simulink model "sm_boom_lift_crawler_abstract"  (R2026a)
settings: Solver=ode23t  StopTime=operator_seq.StopTime  FixedStep=2e-2  MaxStep=2  AbsTol=1e-3
PreLoadFcn:
  | sm_boom_lift_crawler_settest('full test')
StartFcn:
  | tic;
StopFcn:
  | Elapsed_Sim_Time = toc;
  | %disp(['Elapsed Sim Time = ' num2str(Elapsed_Sim_Time)]);
undefined symbols (not defined in the file): BasketR, Boom, Chassis, Extend, Jib, LevelM, LevelS, Lift, operator_seq, OutFL, OutFR, OutRL, OutRR, Tilt, TrackL, TrackR, Turret
libraries: sm_boom_lift_crawler_lib x14, sm_lib x2, sm_boom_lift_crawler_lib_control x1, sm_boom_lift_crawler_lib_lift x1, nesl_utility x1
Description:
  | Boom Lift Crawler with Abstract Actuator Models and Controller
  | 
  | Copyright 2020-2026 The MathWorks, Inc.
settings Model: PacingRate=0.100000  Creator=smiller  LastModifiedBy=smiller
settings DataIOCC: SignalLoggingName=logsout_sm_boom_lift_crawler
settings SimscapeCC: SimscapeNominalValues="[{\"value\":\"1\",\"unit\":\"A\"},{\"value\":\"nomval_psi\",\"unit\":\"psi\"},{\"value\":\"1\",\"unit\":\"cm^2\"},{\"value\":\"nomval_cmv3_s\",\"unit\":\"cm^3/s\"},{\"value\":\"1\",\"unit\":\"kJ/kg\"},{\"value\":\"1\",\"unit\":\"kW\"},{\"value\":\"1\",\"unit\":\"l\"},{\"value\":\"nomval_N\",\"unit\":\"N\"},{\"value\":\"nomval_Nm\",\"unit\":\"N*m\"},{\"value\":\"1\",\"unit\":\"V\"}]"  SimscapeLogName=simlog_sm_boom_lift_crawler  SimscapeLogLimitData=off  SimscapeLogDataHistory=5000.0  SimscapeOperatingPoint=op_hold15Sec_FULL
settings DiagnosticsConfigSet: SimMechanicsConflictingReferenceFrames=none  SimMechanicsRigidlyBoundBlock=none
settings ExplorerConfigSet: InternalSimMechanicsExplorerSettings="<ExplorerConfiguration><canonicalview>default</canonicalview><AnimationSetting><BasePlaybackSpeed>1.0</BasePlaybackSpeed><PlaybackSpeedFactor>4.0</PlaybackSpeedFactor></AnimationSetting><TilePanel><TileInfo><Tiles Columns=\"2\" Count=\"3\" Rows=\"2\"><Column Weight=\"0.4762\"/><Column Weight=\"0.5238\"/><Row Weight=\"0.5\"/><Row Weight=\"0.5\"/><Tile Height=\"1\" Width=\"1\" X=\"0\" Y=\"0\"/><Tile Height=\"1\" Width=\"1\" X=\"0\" Y=\"1\"/><Tile Height=\"2\" Width=\"1\" X=\"1\" Y=\"0\"/></Tiles></TileInfo><SceneInfo><SceneViewer><BGColor><R>1</R><G>1</G><B>1</B></BGColor><Camera><DoPerspective>off</DoPerspective><Position><X>0.0516797948744336932</X><Y>0.487181813254666363</Y><Z>16.9590725690521751</Z></Position><Center><X>0.0516797948744336932</X><Y>0.487181813254666363</Y><Z>1.03715866228651166</Z></Center><Up><X>0.999999952444677764</X><Y>0.000308400133790180664</Y><Z>0</Z></Up><ViewLimDist>1</ViewLimDist><YLim>2.49915112509375037</YLim><XLim>5.22931621973398197</XLim></Camera></SceneViewer><SceneViewer><BGColor><R>1</R><G>1</G><B>1</B></BGColor><Camera><DoPerspective>off</DoPerspective><Position><X>-11.4895183893373876</X><Y>4.05584925644575378e-08</Y><Z>1.89929114001093824</Z></Position><Center><X>-2.67728871072847596e-07</X><Y>4.05584925644575378e-08</Y><Z>1.89929114001093824</Z></Center><Up><X>0</X><Y>0</Y><Z>1</Z></Up><ViewLimDist>1</ViewLimDist><YLim>2.64934859154929603</YLim><XLim>5.54359495206533381</XLim></Camera></SceneViewer><SceneViewer><BGColor><R>1</R><G>1</G><B>1</B></BGColor><Camera><DoPerspective>on</DoPerspective><Position><X>0.00209723334754329926</X><Y>1.29823210500621533</Y><Z>0.569634199895673765</Z></Position><Center><X>0.00166989381543739923</X><Y>2.29823093449923377</Y><Z>0.568165052688056504</Z></Center><Up><X>-0.00271868050236136628</X><Y>0.00146798011384896131</Y><Z>0.999995226893964473</Z></Up><ViewLimDist>1</ViewLimDist><YLim>0.466307658154998583</YLim><XLim>0.530158914250911217</XLim></Camera></SceneViewer></SceneInfo></TilePanel><MechEditorPanel><Cameras><Camera><Id>Camera8</Id><Value><Name>Extend_Knuckle</Name><NativeCamera><PositionTrackingFeature>Lift.Boom.Arms.Telescope.Extend_Cylinder.Transform_Camera_Extend_Knuckle.F</PositionTrackingFeature><CenterTrackingFeature>Lift.Boom.Arms.Telescope.Extend_Cylinder.Transform_Camera_Extend_Knuckle.F</CenterTrackingFeature><UpVectorTrackingFeature>Lift.Boom.Arms.Telescope.Extend_Cylinder.Transform_Camera_Extend_Knuckle.F</UpVectorTrackingFeature><CenterTrackingOrigin>off</CenterTrackingOrigin><CenterTrackingDirection>-X</CenterTrackingDirection><UpVectorTrackingDirection>-Y</UpVectorTrackingDirection></NativeCamera></Value></Camera><Camera><Id>Camera9</Id><Value><Name>Extend_Basket</Name><NativeCamera><PositionTrackingFeature>Lift.Boom.Arms.Telescope.Extend_Cylinder.Transform_Camera_Extend_Basket.F</PositionTrackingFeature><CenterTrackingFeature>Lift.Boom.Arms.Telescope.Extend_Cylinder.Transform_Camera_Extend_Basket.F</CenterTrackingFeature><UpVectorTrackingFeature>Lift.Boom.Arms.Telescope.Extend_Cylinder.Transform_Camera_Extend_Basket.F</UpVectorTrackingFeature><CenterTrackingOrigin>off</CenterTrackingOrigin><CenterTrackingDirection>+X</CenterTrackingDirection><UpVectorTrackingDirection>+Y</UpVectorTrackingDirection></NativeCamera></Value></Camera><Camera><Id>Camera10</Id><Value><Name>Basket_Rotate</Name><NativeCamera><PositionTrackingFeature>Lift.Boom.Basket.Basket_Rotate.Bracket.Reference_Camera_Basket_Rotate_L.R</PositionTrackingFeature><CenterTrackingFeature>Lift.Boom.Basket.Basket_Rotate.Bracket.Reference_Camera_Basket_Rotate_L.R</CenterTrackingFeature><UpVectorTrackingFeature>Mech_Config.World.W</UpVectorTrackingFeature><CenterTrackingOrigin>off</CenterTrackingOrigin><CenterTrackingDirection>-X</CenterTrackingDirection><UpVectorTrackingDirection>+Z</UpVectorTrackingDirection></NativeCamera></Value></Camera><Camera><Id>Camera11</Id><Value><Name>Tilt_Knuckle</Name><NativeCamera><PositionTrackingFeature>Lift.Boom.Arms.Tower.Upper_Knuckle.Reference_Knuckle_Cam.R</PositionTrackingFeature><CenterTrackingFeature>Lift.Boom.Arms.Tower.Upper_Knuckle.Reference_Knuckle_Cam.R</CenterTrackingFeature><UpVectorTrackingFeature>Mech_Config.World.W</UpVectorTrackingFeature><CenterTrackingOrigin>off</CenterTrackingOrigin><CenterTrackingDirection>+Z</CenterTrackingDirection><UpVectorTrackingDirection>+Z</UpVectorTrackingDirection></NativeCamera></Value></Camera><Camera><Id>Camera12</Id><Value><Name>Full Test</Name><NativeCamera><PositionKeyframeSet><Keyframe><Time>0</Time><Value><X>-12.242458171438994</X><Y>-0.1433452642095574</Y><Z>4.1505972342390427</Z></Value></Keyframe><Keyframe><Time>69.026826430124729</Time><Value><X>-14.974593328379619</X><Y>0.0056652615564253064</Y><Z>5.3389029552684786</Z></Value></Keyframe><Keyframe><Time>110.29539843687829</Time><Value><X>-21.00761369699504</X><Y>-0.0057417156870510078</Y><Z>8.0689402037867488</Z></Value></Keyframe><Keyframe><Time>140.70430157635164</Time><Value><X>-31.272784439198116</X><Y>-2.5583130214499052e-10</Y><Z>12.723321478963756</Z></Value></Keyframe><Keyframe><Time>181.77628976806102</Time><Value><X>-31.272784439198116</X><Y>-2.5583130214499052e-10</Y><Z>12.723321478963756</Z></Value></Keyframe><Keyframe><Time>208.0087867386398</Time><Value><X>-23.351505250921551</X><Y>-2.5583182919801497e-10</Y><Z>9.1371534281977738</Z></Value></Keyframe><Keyframe><Time>243.06358572448306</Time><Value><X>-16.577121762622586</X><Y>-2.5583144573665537e-10</Y><Z>6.0702143126734844</Z></Value></Keyframe><Keyframe><Time>273.3415757110605</Time><Value><X>-16.577121762622586</X><Y>-2.5583144573665537e-10</Y><Z>6.0702143126734844</Z></Value></Keyframe><Keyframe><Time>321.2447002217541</Time><Value><X>-13.690590902490033</X><Y>0.01787769923724114</Y><Z>4.7891626503614262</Z></Value></Keyframe><Keyframe><Time>350</Time><Value><X>-13.690590902490033</X><Y>0.01787769923724114</Y><Z>4.7891626503614262</Z></Value></Keyframe></PositionKeyframeSet><CenterKeyframeSet><Keyframe><Time>0</Time><Value><X>-4.621228999686064</X><Y>-0.1433452642095574</Y><Z>4.1505972342390436</Z></Value></Keyframe><Keyframe><Time>69.026826430124729</Time><Value><X>-0.17395018713353672</X><Y>0.0056652615564253064</Y><Z>5.3389029552684786</Z></Value></Keyframe><Keyframe><Time>110.29539843687829</Time><Value><X>-9.0038066291239502</X><Y>-0.0057417156870549491</Y><Z>8.0689402037867524</Z></Value></Keyframe><Keyframe><Time>140.70430157635164</Time><Value><X>-14.136391845814327</X><Y>-2.5583979379462107e-10</Y><Z>12.72332147896376</Z></Value></Keyframe><Keyframe><Time>181.77628976806102</Time><Value><X>-2.3429975002054775</X><Y>-2.5584563781180217e-10</Y><Z>12.723321478963761</Z></Value></Keyframe><Keyframe><Time>208.0087867386398</Time><Value><X>-10.17575261115104</X><Y>-2.5583801743778167e-10</Y><Z>9.1371534281977755</Z></Value></Keyframe><Keyframe><Time>243.06358572448306</Time><Value><X>-0.54476849060194255</X><Y>-2.5583897563257738e-10</Y><Z>6.0702143126734844</Z></Value></Keyframe><Keyframe><Time>273.3415757110605</Time><Value><X>-0.11057247639663359</X><Y>-2.5583917956089291e-10</Y><Z>6.0702143126734844</Z></Value></Keyframe><Keyframe><Time>321.2447002217541</Time><Value><X>-5.3452949964231387</X><Y>0.017877699237237366</Y><Z>4.7891626503614253</Z></Value></Keyframe><Keyframe><Time>350</Time><Value><X>-5.3452949964231387</X><Y>0.017877699237237366</Y><Z>4.7891626503614253</Z></Value></Keyframe></CenterKeyframeSet><UpVectorKeyframeSet><Keyframe><Time>0</Time><Value><X>0</X><Y>0</Y><Z>1</Z></Value></Keyframe><Keyframe><Time>69.026826430124729</Time><Value><X>0</X><Y>0</Y><Z>1</Z></Value></Keyframe><Keyframe><Time>110.29539843687829</Time><Value><X>0</X><Y>0</Y><Z>1</Z></Value></Keyframe><Keyframe><Time>140.70430157635164</Time><Value><X>0</X><Y>0</Y><Z>1</Z></Value></Keyframe><Keyframe><Time>181.77628976806102</Time><Value><X>-2.0731981129868445e-16</X><Y>1.0273382740432149e-31</Y><Z>1</Z></Value></Keyframe><Keyframe><Time>208.0087867386398</Time><Value><X>1.4663775813922931e-57</X><Y>2.9591920320379324e-42</Y><Z>1</Z></Value></Keyframe><Keyframe><Time>243.06358572448306</Time><Value><X>1.3898401336634517e-57</X><Y>2.9591920320379324e-42</Y><Z>1</Z></Value></Keyframe><Keyframe><Time>273.3415757110605</Time><Value><X>1.3898401336605064e-57</X><Y>2.9591920320379324e-42</Y><Z>1</Z></Value></Keyframe><Keyframe><Time>321.2447002217541</Time><Value><X>1.3198478700492623e-57</X><Y>2.9591920320379324e-42</Y><Z>1</Z></Value></Keyframe><Keyframe><Time>350</Time><Value><X>1.0642863113510858e-16</X><Y>-4.813997747953607e-32</Y><Z>1</Z></Value></Keyframe></UpVectorKeyframeSet></NativeCamera></Value></Camera><Camera><Id>Camera13</Id><Value><Name>View_Basket_World</Name><NativeCamera><PositionTrackingFeature>Lift.Boom.Basket.Basket.Reference_Basket_Cam.R</PositionTrackingFeature><CenterTrackingFeature>Mech_Config.World.W</CenterTrackingFeature><UpVectorTrackingFeature>Lift.Boom.Basket.Basket.Reference_Basket_Cam.R</UpVectorTrackingFeature><CenterTrackingOrigin>on</CenterTrackingOrigin><UpVectorTrackingDirection>+Y</UpVectorTrackingDirection></NativeCamera></Value></Camera><Camera><Id>Camera14</Id><Value><Name>View_Worm_Drive</Name><NativeCamera><PositionTrackingFeature>Lift.Boom.Turret.Case.Reference_Worm_Cam.R</PositionTrackingFeature><CenterTrackingFeature>Lift.Boom.Turret.Case.Transform_Worm_Cam.B</CenterTrackingFeature><UpVectorTrackingFeature>Mech_Config.World.W</UpVectorTrackingFeature><CenterTrackingOrigin>on</CenterTrackingOrigin><UpVectorTrackingDirection>+Z</UpVectorTrackingDirection></NativeCamera></Value></Camera><Camera><Id>Camera15</Id><Value><Name>Extend_Retract_Pulley</Name><NativeCamera><PositionTrackingFeature>Lift.Boom.Arms.Telescope.Extend_Cylinder.Reference_Camera_Retract_Pulley.R</PositionTrackingFeature><CenterTrackingFeature>Lift.Boom.Arms.Telescope.Extend_Cylinder.Reference_Camera_Retract_Pulley.R</CenterTrackingFeature><UpVectorTrackingFeature>Lift.Boom.Arms.Telescope.Extend_Cylinder.Reference_Camera_Retract_Pulley.R</UpVectorTrackingFeature><CenterTrackingOrigin>off</CenterTrackingOrigin><CenterTrackingDirection>+Y</CenterTrackingDirection><UpVectorTrackingDirection>+Z</UpVectorTrackingDirection></NativeCamera></Value></Camera><Camera><Id>Camera16</Id><Value><Name>Extend_Extend_Pulley</Name><NativeCamera><PositionTrackingFeature>Lift.Boom.Arms.Telescope.Extend_Cylinder.Reference_Camera_Extend_Pulley.R</PositionTrackingFeature><CenterTrackingFeature>Lift.Boom.Arms.Telescope.Extend_Cylinder.Reference_Camera_Extend_Pulley.R</CenterTrackingFeature><UpVectorTrackingFeature>Lift.Boom.Arms.Telescope.Extend_Cylinder.Reference_Camera_Extend_Pulley.R</UpVectorTrackingFeature><CenterTrackingOrigin>off</CenterTrackingOrigin><CenterTrackingDirection>+Z</CenterTrackingDirection><UpVectorTrackingDirection>-Y</UpVectorTrackingDirection></NativeCamera></Value></Camera><Camera><Id>Camera17</Id><Value><Name>Jib</Name><NativeCamera><PositionTrackingFeature>Lift.Boom.Basket.Jib.Jib_Mount.Reference_Camera_Basket_Jib.R</PositionTrackingFeature><CenterTrackingFeature>Lift.Boom.Basket.Jib.Jib_Mount.Reference_Camera_Basket_Jib.R</CenterTrackingFeature><UpVectorTrackingFeature>Mech_Config.World.W</UpVectorTrackingFeature><CenterTrackingOrigin>off</CenterTrackingOrigin><CenterTrackingDirection>-X</CenterTrackingDirection><UpVectorTrackingDirection>+Z</UpVectorTrackingDirection></NativeCamera></Value></Camera><Camera><Id>Camera18</Id><Value><Name>Boom Align</Name><NativeCamera><PositionTrackingFeature>Lift.Chassis.Frame.Reference_Camera_Boom_Align_R</PositionTrackingFeature><CenterTrackingFeature>Lift.Chassis.Frame.Reference_Camera_Boom_Align_R</CenterTrackingFeature><UpVectorTrackingFeature>Lift.Chassis.Frame.Reference_Camera_Boom_Align_R</UpVectorTrackingFeature><CenterTrackingOrigin>off</CenterTrackingOrigin><CenterTrackingDirection>+Y</CenterTrackingDirection><UpVectorTrackingDirection>+Z</UpVectorTrackingDirection></NativeCamera></Value></Camera><Camera><Id>Camera19</Id><Value><Name>Basket Boom</Name><NativeCamera><PositionTrackingFeature>Lift.Boom.Arms.Camera_Basket_Boom.Reference_Basket_Boom_Cam.R</PositionTrackingFeature><CenterTrackingFeature>Lift.Boom.Arms.Camera_Basket_Boom.Reference_Basket_Boom_Cam.R</CenterTrackingFeature><UpVectorTrackingFeature>Mech_Config.World.W</UpVectorTrackingFeature><CenterTrackingOrigin>off</CenterTrackingOrigin><CenterTrackingDirection>+Y</CenterTrackingDirection><UpVectorTrackingDirection>+Z</UpVectorTrackingDirection></NativeCamera></Value></Camera></Cameras><GfxPanelCameraMap><MapElement CameraMLId=\"Camera18\" GfxPanelIndex=\"2\"/></GfxPanelCameraMap><VideoCreator><PlaybackSpeedRatio>0.25</PlaybackSpeedRatio><FrameRate>30</FrameRate><VideoFormat>MPEG-4</VideoFormat><FrameSize>auto</FrameSize></VideoCreator></MechEditorPanel></ExplorerConfiguration>"

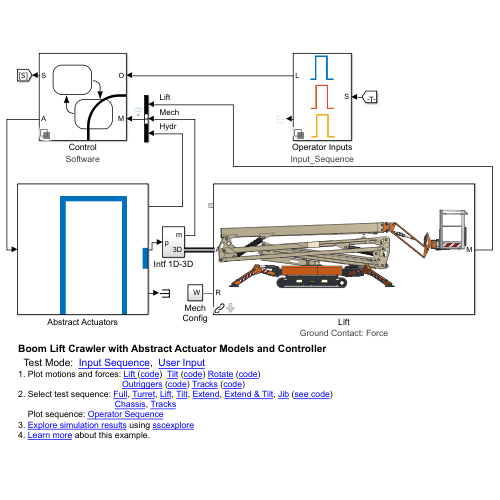
[thumbnail: Simulink's stored preview of the top-level diagram]
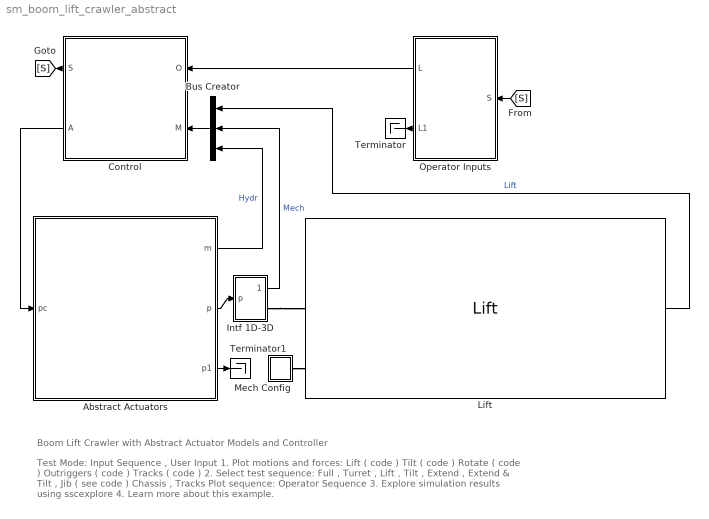
== system sm_boom_lift_crawler_abstract ==
  note: Test Mode: Input Sequence , User Input
      | 1. Plot motions and forces: Lift ( code ) Tilt ( code ) Rotate ( code )
      | Outriggers ( code ) Tracks ( code )
      | 2. Select test sequence: Full , Turret , Lift , Tilt , Extend , Extend & Tilt , Jib ( see code )
      | Chassis , Tracks
      | Plot sequence: Operator Sequence
      | 3. Explore simulation results using sscexplore
      | 4. Learn more about this example.
  note: Boom Lift Crawler with Abstract Actuator Models and Controller
  Abstract Actuators : Subsystem  VariantControl=Controller_Inputs
      mask Display: image('sm_boom_lift_crawler_logic_to_motion_seq.svg');
  Bus Creator : BusCreator  Inputs=3
  Control : Subsystem  Variant=on  VariantControlMode=label  VariantControl=Variant1  LabelModeActiveChoice=Software
      settings: AttributesFormatString=%<LabelModeActiveChoice>
      mask Display:
      | blk = sm_boom_lift_activeVariantBlock(gcb);
      | eval(get_param(blk, 'MaskDisplay'));
  Intf 1D-3D : Subsystem
  Lift : sm_boom_lift_crawler_lib_lift/Lift  popup_gnd_outr=Force
      settings: AttributesFormatString=Ground Contact: %<popup_gnd_outr>
  Mech Config : Subsystem
  Operator Inputs : Subsystem  Variant=on  VariantControlMode=label  VariantControl=Variant1  LabelModeActiveChoice=Input_Sequence
      settings: AttributesFormatString=%<LabelModeActiveChoice>
      mask Display:
      | blk = sm_boom_lift_activeVariantBlock(gcb);
      | eval(get_param(blk, 'MaskDisplay'));
  Terminator : Terminator
  Terminator1 : Terminator
  wires:
  Intf 1D-3D/1(m) -> Bus Creator/2  "Mech"
  Bus Creator/1 -> Control/2(M)
  Lift/1 -> Bus Creator/1  "Lift"
  Control/2(A) -> Abstract Actuators/1(pc)
  Abstract Actuators/2(p) -> Intf 1D-3D/1(p)
  Abstract Actuators/3(p1) -> Terminator1/1
  Abstract Actuators/1(m) -> Bus Creator/3  "Hydr"
  Operator Inputs/1(L) -> Control/1(O)
  Operator Inputs/2(L1) -> Terminator/1
  Control/1(S) -> [S]
  [S] -> Operator Inputs/1(S)
  connections:
  Mech Config/LConn1 -- Lift/LConn3
  Intf 1D-3D/RConn1 -- Lift/LConn2

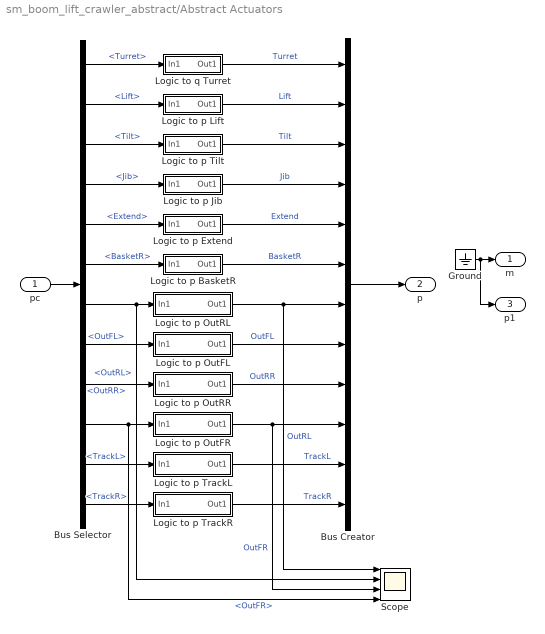
== system sm_boom_lift_crawler_abstract/Abstract Actuators ==
  pc : Inport
  Bus Creator : BusCreator  Inputs=12
  Bus Selector : BusSelector  OutputSignals=Turret,Lift,Tilt,Jib,Extend,BasketR,OutRL,OutFL,OutRR,OutFR,TrackL,TrackR
  Ground : Ground
  Logic to p BasketR : Subsystem
  Logic to p Extend : Subsystem
  Logic to p Jib : Subsystem
  Logic to p Lift : Subsystem
  Logic to p OutFL : Subsystem
  Logic to p OutFR : Subsystem
  Logic to p OutRL : Subsystem
  Logic to p OutRR : Subsystem
  Logic to p Tilt : Subsystem
  Logic to p TrackL : Subsystem
  Logic to p TrackR : Subsystem
  Logic to q Turret : Subsystem
  Scope : Scope  NumInputPorts=4
      settings: ActiveDisplayYMinimum=12.92005  ActiveDisplayYMaximum=13.76598
  m : Outport
  p : Outport  Port=2
  p1 : Outport  Port=3
  wires:
  Ground/1 -> m/1, p1/1
  pc/1 -> Bus Selector/1
  Bus Selector/12 -> Logic to p TrackR/1(In1)  "<TrackR>"
  Bus Selector/11 -> Logic to p TrackL/1(In1)  "<TrackL>"
  Bus Selector/2 -> Logic to p Lift/1(In1)  "<Lift>"
  Logic to p TrackL/1(Out1) -> Bus Creator/11  "TrackL"
  Bus Selector/6 -> Logic to p BasketR/1(In1)  "<BasketR>"
  Bus Selector/5 -> Logic to p Extend/1(In1)  "<Extend>"
  Bus Creator/1 -> p/1
  Bus Selector/1 -> Logic to q Turret/1(In1)  "<Turret>"
  Bus Selector/7 -> Scope/2, Logic to p OutRL/1(In1)  "<OutRL>"
  Bus Selector/3 -> Logic to p Tilt/1(In1)  "<Tilt>"
  Logic to p Lift/1(Out1) -> Bus Creator/2  "Lift"
  Bus Selector/8 -> Logic to p OutFL/1(In1)  "<OutFL>"
  Bus Selector/4 -> Logic to p Jib/1(In1)  "<Jib>"
  Logic to p TrackR/1(Out1) -> Bus Creator/12  "TrackR"
  Bus Selector/9 -> Logic to p OutRR/1(In1)  "<OutRR>"
  Bus Selector/10 -> Scope/4, Logic to p OutFR/1(In1)  "<OutFR>"
  Logic to q Turret/1(Out1) -> Bus Creator/1  "Turret"
  Logic to p OutRL/1(Out1) -> Scope/1, Bus Creator/7  "OutRL"
  Logic to p OutFL/1(Out1) -> Bus Creator/8  "OutFL"
  Logic to p OutRR/1(Out1) -> Bus Creator/9  "OutRR"
  Logic to p OutFR/1(Out1) -> Scope/3, Bus Creator/10  "OutFR"
  Logic to p Tilt/1(Out1) -> Bus Creator/3  "Tilt"
  Logic to p Jib/1(Out1) -> Bus Creator/4  "Jib"
  Logic to p Extend/1(Out1) -> Bus Creator/5  "Extend"
  Logic to p BasketR/1(Out1) -> Bus Creator/6  "BasketR"

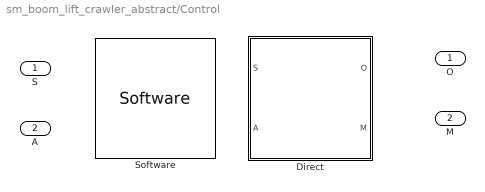
== system sm_boom_lift_crawler_abstract/Control ==
  O : Inport
  M : Inport  Port=2
  Direct : Subsystem  VariantControl=Direct
      mask Display: image('sm_boom_lift_crawler_control_direct.svg');
  Software : sm_boom_lift_crawler_lib_control/Software  SystemSampleTime=-1  VariantControl=Software  VariantActivationTime=update diagram  EmptyChoice=off  PassThrough=off  PassThroughVariantControl=(default)  EmptyChoiceVariantControl=(default)  AllowFlexibleInterface=on  Latency=0  AutoFrameSizeCalculation=off
  S : Outport
  A : Outport  Port=2

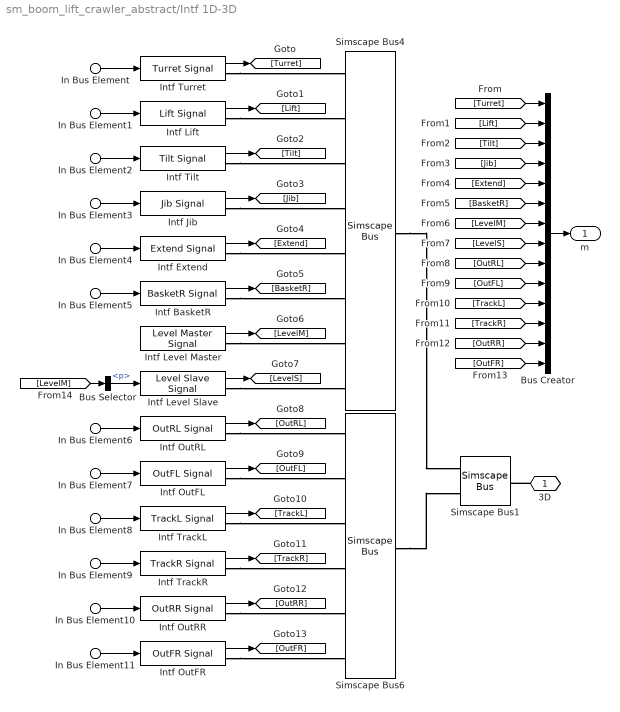
== system sm_boom_lift_crawler_abstract/Intf 1D-3D ==
  In Bus Element : Inport  PortName=p  Element=Turret
  In Bus Element1 : Inport  PortName=p  Element=Lift
  In Bus Element2 : Inport  PortName=p  Element=Tilt
  In Bus Element3 : Inport  PortName=p  Element=Jib
  In Bus Element4 : Inport  PortName=p  Element=Extend
  In Bus Element5 : Inport  PortName=p  Element=BasketR
  In Bus Element6 : Inport  PortName=p  Element=OutRL
  In Bus Element7 : Inport  PortName=p  Element=OutFL
  In Bus Element8 : Inport  PortName=p  Element=TrackL
  In Bus Element9 : Inport  PortName=p  Element=TrackR
  In Bus Element10 : Inport  PortName=p  Element=OutRR
  In Bus Element11 : Inport  PortName=p  Element=OutFR
  Bus Creator : BusCreator  Inputs=14
  Bus Selector : BusSelector  OutputSignals=p
  Intf BasketR : sm_boom_lift_crawler_lib/BasketR Signal  SystemSampleTime=-1  VariantActivationTime=update diagram  EmptyChoice=off  PassThrough=off  PassThroughVariantControl=(default)  EmptyChoiceVariantControl=(default)  AllowFlexibleInterface=on  Latency=0  AutoFrameSizeCalculation=off
  Intf Extend : sm_boom_lift_crawler_lib/Extend Signal  SystemSampleTime=-1  VariantActivationTime=update diagram  EmptyChoice=off  PassThrough=off  PassThroughVariantControl=(default)  EmptyChoiceVariantControl=(default)  AllowFlexibleInterface=on  Latency=0  AutoFrameSizeCalculation=off
  Intf Jib : sm_boom_lift_crawler_lib/Jib Signal  SystemSampleTime=-1  VariantActivationTime=update diagram  EmptyChoice=off  PassThrough=off  PassThroughVariantControl=(default)  EmptyChoiceVariantControl=(default)  AllowFlexibleInterface=on  Latency=0  AutoFrameSizeCalculation=off
  Intf Level Master : sm_boom_lift_crawler_lib/Level Master Signal  SystemSampleTime=-1  VariantActivationTime=update diagram  EmptyChoice=off  PassThrough=off  PassThroughVariantControl=(default)  EmptyChoiceVariantControl=(default)  AllowFlexibleInterface=on  Latency=0  AutoFrameSizeCalculation=off
  Intf Level Slave : sm_boom_lift_crawler_lib/Level Slave Signal  SystemSampleTime=-1  VariantActivationTime=update diagram  EmptyChoice=off  PassThrough=off  PassThroughVariantControl=(default)  EmptyChoiceVariantControl=(default)  AllowFlexibleInterface=on  Latency=0  AutoFrameSizeCalculation=off
  Intf Lift : sm_boom_lift_crawler_lib/Lift Signal  SystemSampleTime=-1  VariantActivationTime=update diagram  EmptyChoice=off  PassThrough=off  PassThroughVariantControl=(default)  EmptyChoiceVariantControl=(default)  AllowFlexibleInterface=on  Latency=0  AutoFrameSizeCalculation=off
  Intf OutFL : sm_boom_lift_crawler_lib/OutFL Signal  SystemSampleTime=-1  VariantActivationTime=update diagram  EmptyChoice=off  PassThrough=off  PassThroughVariantControl=(default)  EmptyChoiceVariantControl=(default)  AllowFlexibleInterface=on  Latency=0  AutoFrameSizeCalculation=off
  Intf OutFR : sm_boom_lift_crawler_lib/OutFR Signal  SystemSampleTime=-1  VariantActivationTime=update diagram  EmptyChoice=off  PassThrough=off  PassThroughVariantControl=(default)  EmptyChoiceVariantControl=(default)  AllowFlexibleInterface=on  Latency=0  AutoFrameSizeCalculation=off
  Intf OutRL : sm_boom_lift_crawler_lib/OutRL Signal  SystemSampleTime=-1  VariantActivationTime=update diagram  EmptyChoice=off  PassThrough=off  PassThroughVariantControl=(default)  EmptyChoiceVariantControl=(default)  AllowFlexibleInterface=on  Latency=0  AutoFrameSizeCalculation=off
  Intf OutRR : sm_boom_lift_crawler_lib/OutRR Signal  SystemSampleTime=-1  VariantActivationTime=update diagram  EmptyChoice=off  PassThrough=off  PassThroughVariantControl=(default)  EmptyChoiceVariantControl=(default)  AllowFlexibleInterface=on  Latency=0  AutoFrameSizeCalculation=off
  Intf Tilt : sm_boom_lift_crawler_lib/Tilt Signal  SystemSampleTime=-1  VariantActivationTime=update diagram  EmptyChoice=off  PassThrough=off  PassThroughVariantControl=(default)  EmptyChoiceVariantControl=(default)  AllowFlexibleInterface=on  Latency=0  AutoFrameSizeCalculation=off
  Intf TrackL : sm_boom_lift_crawler_lib/TrackL Signal  SystemSampleTime=-1  VariantActivationTime=update diagram  EmptyChoice=off  PassThrough=off  PassThroughVariantControl=(default)  EmptyChoiceVariantControl=(default)  AllowFlexibleInterface=on  Latency=0  AutoFrameSizeCalculation=off
  Intf TrackR : sm_boom_lift_crawler_lib/TrackR Signal  SystemSampleTime=-1  VariantActivationTime=update diagram  EmptyChoice=off  PassThrough=off  PassThroughVariantControl=(default)  EmptyChoiceVariantControl=(default)  AllowFlexibleInterface=on  Latency=0  AutoFrameSizeCalculation=off
  Intf Turret : sm_boom_lift_crawler_lib/Turret Signal  SystemSampleTime=-1  VariantActivationTime=update diagram  EmptyChoice=off  PassThrough=off  PassThroughVariantControl=(default)  EmptyChoiceVariantControl=(default)  AllowFlexibleInterface=on  Latency=0  AutoFrameSizeCalculation=off
  Simscape Bus1 : SimscapeBus  HierarchyStrings=Boom;Chassis
  Simscape Bus4 : SimscapeBus  HierarchyStrings=Turret;Lift;Tilt;Jib;Extend;BasketR;LevelM;LevelS
  Simscape Bus6 : SimscapeBus  HierarchyStrings=OutRL;OutFL;TrackL;TrackR;OutRR;OutFR
  3D : PMIOPort  Side=Right
  m : Outport
  wires:
  Intf OutFR/1 -> [OutFR]
  Intf OutRR/1 -> [OutRR]
  Intf TrackR/1 -> [TrackR]
  Intf TrackL/1 -> [TrackL]
  Intf OutFL/1 -> [OutFL]
  Intf OutRL/1 -> [OutRL]
  Intf Level Slave/1 -> [LevelS]
  Intf Level Master/1 -> [LevelM]
  Intf BasketR/1 -> [BasketR]
  Intf Extend/1 -> [Extend]
  Intf Jib/1 -> [Jib]
  Intf Tilt/1 -> [Tilt]
  Intf Lift/1 -> [Lift]
  Intf Turret/1 -> [Turret]
  [OutFR] -> Bus Creator/14
  [OutRR] -> Bus Creator/13
  [Extend] -> Bus Creator/5
  [OutRL] -> Bus Creator/9
  [TrackL] -> Bus Creator/11
  [LevelM] -> Bus Creator/7
  [Turret] -> Bus Creator/1
  [OutFL] -> Bus Creator/10
  [Tilt] -> Bus Creator/3
  [Lift] -> Bus Creator/2
  [TrackR] -> Bus Creator/12
  [LevelS] -> Bus Creator/8
  Bus Creator/1 -> m/1
  [Jib] -> Bus Creator/4
  [BasketR] -> Bus Creator/6
  Bus Selector/1 -> Intf Level Slave/1  "<p>"
  [LevelM] -> Bus Selector/1
  In Bus Element/1 -> Intf Turret/1
  In Bus Element1/1 -> Intf Lift/1
  In Bus Element2/1 -> Intf Tilt/1
  In Bus Element3/1 -> Intf Jib/1
  In Bus Element4/1 -> Intf Extend/1
  In Bus Element5/1 -> Intf BasketR/1
  In Bus Element6/1 -> Intf OutRL/1
  In Bus Element7/1 -> Intf OutFL/1
  In Bus Element8/1 -> Intf TrackL/1
  In Bus Element9/1 -> Intf TrackR/1
  In Bus Element10/1 -> Intf OutRR/1
  In Bus Element11/1 -> Intf OutFR/1
  connections:
  Intf OutRR/RConn1 -- Simscape Bus6/LConn5
  Intf OutFR/RConn1 -- Simscape Bus6/LConn6
  Intf TrackR/RConn1 -- Simscape Bus6/LConn4
  Intf TrackL/RConn1 -- Simscape Bus6/LConn3
  Intf OutRL/RConn1 -- Simscape Bus6/LConn1
  Intf OutFL/RConn1 -- Simscape Bus6/LConn2
  Simscape Bus6/RConn1 -- Simscape Bus1/LConn2
  Intf Level Slave/RConn1 -- Simscape Bus4/LConn8
  Intf Level Master/RConn1 -- Simscape Bus4/LConn7
  Intf BasketR/RConn1 -- Simscape Bus4/LConn6
  Intf Extend/RConn1 -- Simscape Bus4/LConn5
  Intf Jib/RConn1 -- Simscape Bus4/LConn4
  Intf Tilt/RConn1 -- Simscape Bus4/LConn3
  Intf Lift/RConn1 -- Simscape Bus4/LConn2
  Intf Turret/RConn1 -- Simscape Bus4/LConn1
  Simscape Bus4/RConn1 -- Simscape Bus1/LConn1
  3D/RConn1 -- Simscape Bus1/RConn1

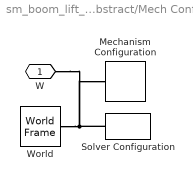
== system sm_boom_lift_crawler_abstract/Mech Config ==
  Mechanism Configuration : sm_lib/Utilities/Mechanism Configuration  UniformGravity=Constant  GravityVector=[0 0 -9.80665]  GravityVectorUnits=m/s^2  LinearizationDelta=0.001  JointModeTransitionNonlinearIterations=2
  Solver Configuration : nesl_utility/Solver Configuration  PhysicalDomain=network_engine_domain  SubClassName=solver  LeftPortType=input  RightPortType=generic  Tones=[]  Harmonics=[]  SimulateNoise=off  Profile=off  UseLocalSampling=off  EnableSwitchedLinearOptims=on  FrequencyDomain=off  UseCCode=off  RelTol=0.001  AbsTol=1e-06  MinStep=1e-09  ToWorkspace=off  RevertToSquareIcSolve=off  NumHomotopyIterations=100  PhasorMode=off  PhasorModeNumHarmonics=1  ConsistencySolver=NEWTON_FTOL  CanonicalOrdering=UNORDERED  OptimizeIntermediates=UNOPTIMIZED  IndexReductionMethod=DerivativeReplacement  DoDC=off  ResidualTolerance=1e-9  ConsistencyTolSource=GLOBAL  ConsistencyAbsTol=0.001  ConsistencyRelTol=0.001  ConsistencyTolFactor=0.001  UseLocalSolver=off  LocalSolverChoice=NE_BACKWARD_EULER_ADVANCER  ResolveIndetEquations=on  FunctionEvalNumThread=1  LocalSolverSampleTime=2e-3  DoFixedCost=off  MaxNonlinIter=3  MaxModeIter=2  ComputeImpulses=off  ImpulseIterations=2  LinearAlgebra=auto  LinearAlgebraNumThread=0  EquationFormulation=NE_TIME_EF  DelaysMemoryBudget=1024  AutomaticFiltering=on  FilteringTimeConstant=0.001  PartitionStorageMethod=AS_NEEDED  PartitionMemoryBudget=1024  PartitionMethod=ROBUST  MultibodyUseLocalSolver=off  MultibodyLocalSolverChoice=ODE1  MultibodyLocalSolverSampleTime=0.001
  World : sm_lib/Frames and Transforms/World Frame
  W : PMIOPort  Side=Left
  connections:
  Solver Configuration/RConn1 -- W/RConn1 -- Mechanism Configuration/RConn1 -- World/RConn1

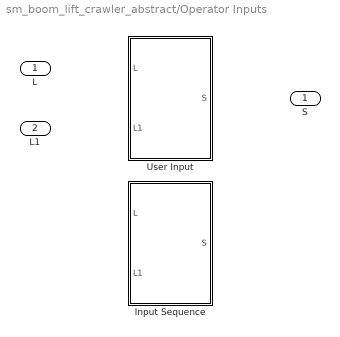
== system sm_boom_lift_crawler_abstract/Operator Inputs ==
  S : Inport
  Input Sequence : Subsystem  VariantControl=Input_Sequence
      mask Display: image('sm_boom_lift_crawler_operator_seq.svg');
  User Input : Subsystem  VariantControl=User_Input
      mask Display: image('sl001_2x3.svg');
  L : Outport
  L1 : Outport  Port=2

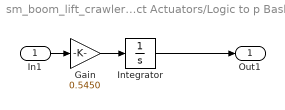
== system sm_boom_lift_crawler_abstract/Abstract Actuators/Logic to p BasketR ==
  In1 : Inport
  Gain : Gain  Gain=0.5450
  Integrator : Integrator  LimitOutput=on  UpperSaturationLimit=1.09  LowerSaturationLimit=0
  Out1 : Outport
  wires:
  Gain/1 -> Integrator/1
  In1/1 -> Gain/1
  Integrator/1 -> Out1/1

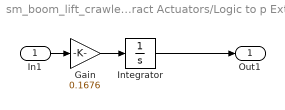
== system sm_boom_lift_crawler_abstract/Abstract Actuators/Logic to p Extend ==
  In1 : Inport
  Gain : Gain  Gain=0.1676
  Integrator : Integrator  InitialCondition=0.0063  LimitOutput=on  UpperSaturationLimit=3.86  LowerSaturationLimit=0
  Out1 : Outport
  wires:
  Integrator/1 -> Out1/1
  In1/1 -> Gain/1
  Gain/1 -> Integrator/1

== system sm_boom_lift_crawler_abstract/Abstract Actuators/Logic to p Jib ==
  In1 : Inport
  Gain : Gain  Gain=0.0373
  Integrator : Integrator  LimitOutput=on  UpperSaturationLimit=0.358  LowerSaturationLimit=0
  Out1 : Outport
  wires:
  Gain/1 -> Integrator/1
  In1/1 -> Gain/1
  Integrator/1 -> Out1/1

== system sm_boom_lift_crawler_abstract/Abstract Actuators/Logic to p Lift ==
  In1 : Inport
  Gain : Gain  Gain=0.0120
  Integrator : Integrator  LimitOutput=on  UpperSaturationLimit=0.57  LowerSaturationLimit=0
  Out1 : Outport
  wires:
  Gain/1 -> Integrator/1
  In1/1 -> Gain/1
  Integrator/1 -> Out1/1

== system sm_boom_lift_crawler_abstract/Abstract Actuators/Logic to p OutFL ==
  In1 : Inport
  Gain : Gain  Gain=0.2951
  Integrator : Integrator  InitialCondition=13.359685039370081  LimitOutput=on  UpperSaturationLimit=15.07125  LowerSaturationLimit=10
  Out1 : Outport
  wires:
  In1/1 -> Gain/1
  Gain/1 -> Integrator/1
  Integrator/1 -> Out1/1

== system sm_boom_lift_crawler_abstract/Abstract Actuators/Logic to p OutFR ==
  In1 : Inport
  Gain : Gain  Gain=0.2951
  Integrator : Integrator  InitialCondition=13.359685039370081  LimitOutput=on  UpperSaturationLimit=15.07125  LowerSaturationLimit=10
  Out1 : Outport
  wires:
  Gain/1 -> Integrator/1
  In1/1 -> Gain/1
  Integrator/1 -> Out1/1

== system sm_boom_lift_crawler_abstract/Abstract Actuators/Logic to p OutRL ==
  In1 : Inport
  Gain : Gain  Gain=0.2917
  Integrator : Integrator  InitialCondition=13.004645669291337  LimitOutput=on  UpperSaturationLimit=14.69659  LowerSaturationLimit=10
  Out1 : Outport
  wires:
  Gain/1 -> Integrator/1
  In1/1 -> Gain/1
  Integrator/1 -> Out1/1

== system sm_boom_lift_crawler_abstract/Abstract Actuators/Logic to p OutRR ==
  In1 : Inport
  Gain : Gain  Gain=0.2911
  Integrator : Integrator  InitialCondition=13.207637795275589  LimitOutput=on  UpperSaturationLimit=14.89625  LowerSaturationLimit=10
  Out1 : Outport
  wires:
  Gain/1 -> Integrator/1
  In1/1 -> Gain/1
  Integrator/1 -> Out1/1

== system sm_boom_lift_crawler_abstract/Abstract Actuators/Logic to p Tilt ==
  In1 : Inport
  Gain : Gain  Gain=0.0139
  Integrator : Integrator  LimitOutput=on  UpperSaturationLimit=0.57  LowerSaturationLimit=0
  Out1 : Outport
  wires:
  Integrator/1 -> Out1/1
  In1/1 -> Gain/1
  Gain/1 -> Integrator/1

== system sm_boom_lift_crawler_abstract/Abstract Actuators/Logic to p TrackL ==
  In1 : Inport
  Gain : Gain  Gain=1/7
  Integrator : Integrator  LimitOutput=on  UpperSaturationLimit=0.305  LowerSaturationLimit=0
  Out1 : Outport
  wires:
  In1/1 -> Gain/1
  Integrator/1 -> Out1/1
  Gain/1 -> Integrator/1

== system sm_boom_lift_crawler_abstract/Abstract Actuators/Logic to p TrackR ==
  In1 : Inport
  Gain : Gain  Gain=1/7
  Integrator : Integrator  LimitOutput=on  UpperSaturationLimit=0.305  LowerSaturationLimit=0
  Out1 : Outport
  wires:
  Gain/1 -> Integrator/1
  Integrator/1 -> Out1/1
  In1/1 -> Gain/1

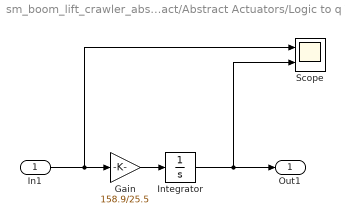
== system sm_boom_lift_crawler_abstract/Abstract Actuators/Logic to q Turret ==
  In1 : Inport
  Gain : Gain  Gain=158.9/25.5
  Integrator : Integrator  LimitOutput=on  UpperSaturationLimit=158.9  LowerSaturationLimit=-158.9
  Scope : Scope  NumInputPorts=2
      settings: ActiveDisplayYMinimum=-1.25  ActiveDisplayYMaximum=1.25  DataLoggingVariableName=ScopeData3
  Out1 : Outport
  wires:
  Integrator/1 -> Scope/2, Out1/1
  In1/1 -> Scope/1, Gain/1
  Gain/1 -> Integrator/1

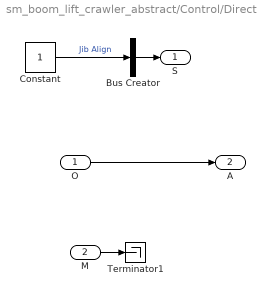
== system sm_boom_lift_crawler_abstract/Control/Direct ==
  O : Inport
  M : Inport  Port=2
  Bus Creator : BusCreator  Inputs=1
  Constant : Constant
  Terminator1 : Terminator
  S : Outport
  A : Outport  Port=2
  wires:
  M/1 -> Terminator1/1
  O/1 -> A/1
  Bus Creator/1 -> S/1
  Constant/1 -> Bus Creator/1  "Jib Align"

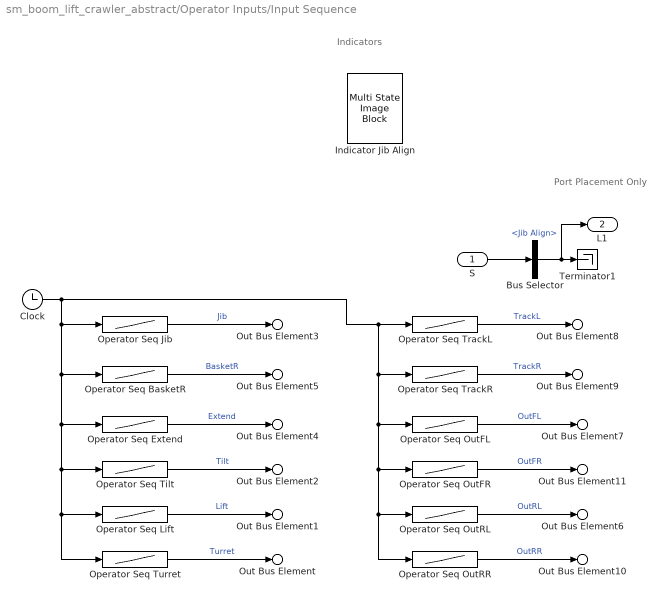
== system sm_boom_lift_crawler_abstract/Operator Inputs/Input Sequence ==
  note: Indicators
  note: Port
      | Placement
      | Only
  S : Inport
  Bus Selector : BusSelector  OutputSignals=Jib Align
  Clock : Clock
  Indicator Jib Align : MultiStateImageBlock
  Operator Seq BasketR : Lookup_n-D  NumberOfTableDimensions=1  BreakpointsForDimension1=operator_seq.basketR.t  Table=operator_seq.basketR.q  InterpMethod=Flat  ExtrapMethod=Clip  UseLastTableValue=on  InternalRulePriority=Speed  RndMeth=Simplest
  Operator Seq Extend : Lookup_n-D  NumberOfTableDimensions=1  BreakpointsForDimension1=operator_seq.extend.t  Table=operator_seq.extend.p  InterpMethod=Flat  ExtrapMethod=Clip  UseLastTableValue=on  InternalRulePriority=Speed  RndMeth=Simplest
  Operator Seq Jib : Lookup_n-D  NumberOfTableDimensions=1  BreakpointsForDimension1=operator_seq.jib.t  Table=operator_seq.jib.p  InterpMethod=Flat  ExtrapMethod=Clip  UseLastTableValue=on  InternalRulePriority=Speed  RndMeth=Simplest
  Operator Seq Lift : Lookup_n-D  NumberOfTableDimensions=1  BreakpointsForDimension1=operator_seq.lift.t  Table=operator_seq.lift.p  InterpMethod=Flat  ExtrapMethod=Clip  UseLastTableValue=on  InternalRulePriority=Speed  RndMeth=Simplest
  Operator Seq OutFL : Lookup_n-D  NumberOfTableDimensions=1  BreakpointsForDimension1=operator_seq.outFL.t  Table=operator_seq.outFL.p  InterpMethod=Flat  ExtrapMethod=Clip  UseLastTableValue=on  InternalRulePriority=Speed  RndMeth=Simplest
  Operator Seq OutFR : Lookup_n-D  NumberOfTableDimensions=1  BreakpointsForDimension1=operator_seq.outFR.t  Table=operator_seq.outFR.p  InterpMethod=Flat  ExtrapMethod=Clip  UseLastTableValue=on  InternalRulePriority=Speed  RndMeth=Simplest
  Operator Seq OutRL : Lookup_n-D  NumberOfTableDimensions=1  BreakpointsForDimension1=operator_seq.outRL.t  Table=operator_seq.outRL.p  InterpMethod=Flat  ExtrapMethod=Clip  UseLastTableValue=on  InternalRulePriority=Speed  RndMeth=Simplest
  Operator Seq OutRR : Lookup_n-D  NumberOfTableDimensions=1  BreakpointsForDimension1=operator_seq.outRR.t  Table=operator_seq.outRR.p  InterpMethod=Flat  ExtrapMethod=Clip  UseLastTableValue=on  InternalRulePriority=Speed  RndMeth=Simplest
  Operator Seq Tilt : Lookup_n-D  NumberOfTableDimensions=1  BreakpointsForDimension1=operator_seq.tilt.t  Table=operator_seq.tilt.p  InterpMethod=Flat  ExtrapMethod=Clip  UseLastTableValue=on  InternalRulePriority=Speed  RndMeth=Simplest
  Operator Seq TrackL : Lookup_n-D  NumberOfTableDimensions=1  BreakpointsForDimension1=operator_seq.TrackL.t  Table=operator_seq.TrackL.p  InterpMethod=Flat  ExtrapMethod=Clip  UseLastTableValue=on  InternalRulePriority=Speed  RndMeth=Simplest
  Operator Seq TrackR : Lookup_n-D  NumberOfTableDimensions=1  BreakpointsForDimension1=operator_seq.TrackR.t  Table=operator_seq.TrackR.p  InterpMethod=Flat  ExtrapMethod=Clip  UseLastTableValue=on  InternalRulePriority=Speed  RndMeth=Simplest
  Operator Seq Turret : Lookup_n-D  NumberOfTableDimensions=1  BreakpointsForDimension1=operator_seq.turret.t  Table=operator_seq.turret.q  InterpMethod=Flat  ExtrapMethod=Clip  UseLastTableValue=on  InternalRulePriority=Speed  RndMeth=Simplest
  Terminator1 : Terminator
  Out Bus Element : Outport  PortName=L  Element=Turret
  Out Bus Element1 : Outport  PortName=L  Element=Lift
  Out Bus Element2 : Outport  PortName=L  Element=Tilt
  Out Bus Element3 : Outport  PortName=L  Element=Jib
  Out Bus Element4 : Outport  PortName=L  Element=Extend
  Out Bus Element5 : Outport  PortName=L  Element=BasketR
  Out Bus Element6 : Outport  PortName=L  Element=OutRL
  Out Bus Element7 : Outport  PortName=L  Element=OutFL
  Out Bus Element8 : Outport  PortName=L  Element=TrackL
  Out Bus Element9 : Outport  PortName=L  Element=TrackR
  Out Bus Element10 : Outport  PortName=L  Element=OutRR
  Out Bus Element11 : Outport  PortName=L  Element=OutFR
  L1 : Outport  Port=2
  wires:
  Operator Seq TrackR/1 -> Out Bus Element9/1  "TrackR"
  Bus Selector/1 -> Terminator1/1, L1/1  "<Jib Align>"
  S/1 -> Bus Selector/1
  Operator Seq Extend/1 -> Out Bus Element4/1  "Extend"
  Operator Seq Turret/1 -> Out Bus Element/1  "Turret"
  Operator Seq Lift/1 -> Out Bus Element1/1  "Lift"
  Operator Seq Tilt/1 -> Out Bus Element2/1  "Tilt"
  Operator Seq OutFL/1 -> Out Bus Element7/1  "OutFL"
  Operator Seq BasketR/1 -> Out Bus Element5/1  "BasketR"
  Operator Seq Jib/1 -> Out Bus Element3/1  "Jib"
  Operator Seq OutRL/1 -> Out Bus Element6/1  "OutRL"
  Operator Seq OutFR/1 -> Out Bus Element11/1  "OutFR"
  Operator Seq OutRR/1 -> Out Bus Element10/1  "OutRR"
  Operator Seq TrackL/1 -> Out Bus Element8/1  "TrackL"
  Clock/1 -> Operator Seq TrackR/1, Operator Seq OutFL/1, Operator Seq OutFR/1, Operator Seq OutRL/1, Operator Seq OutRR/1, Operator Seq TrackL/1, Operator Seq Jib/1, Operator Seq BasketR/1, Operator Seq Extend/1, Operator Seq Tilt/1, Operator Seq Lift/1, Operator Seq Turret/1

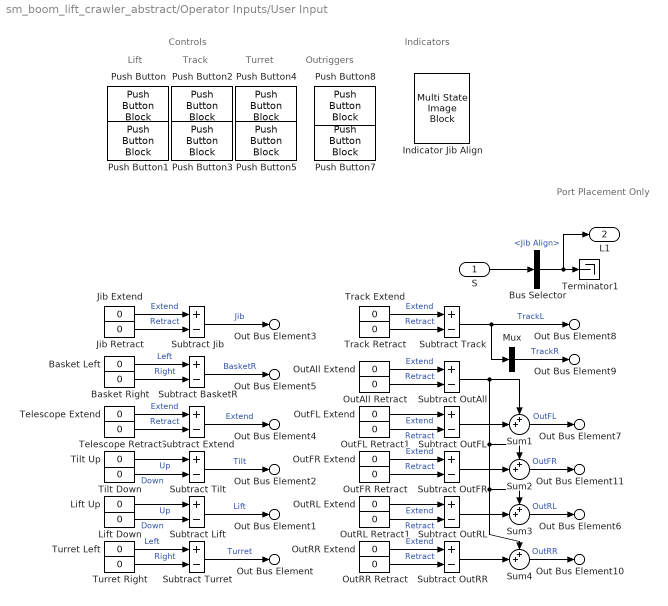
== system sm_boom_lift_crawler_abstract/Operator Inputs/User Input ==
  note: Controls
  note: Lift
  note: Port
      | Placement
      | Only
  note: Track
  note: Turret
  note: Indicators
  note: Outriggers
  S : Inport
  Basket Left : Constant  Value=0
  Basket Right : Constant  Value=0
  Bus Selector : BusSelector  OutputSignals=Jib Align
  Indicator Jib Align : MultiStateImageBlock
  Jib Extend : Constant  Value=0
  Jib Retract : Constant  Value=0
  Lift Down : Constant  Value=0
  Lift Up : Constant  Value=0
  Mux : Mux  Inputs=1
  OutAll Extend : Constant  Value=0
  OutAll Retract : Constant  Value=0
  OutFL Extend : Constant  Value=0
  OutFL Retract1 : Constant  Value=0
  OutFR Extend : Constant  Value=0
  OutFR Retract : Constant  Value=0
  OutRL Extend : Constant  Value=0
  OutRL Retract1 : Constant  Value=0
  OutRR Extend : Constant  Value=0
  OutRR Retract : Constant  Value=0
  Push Button : PushButtonBlock  ButtonText=Up  IconOnColor=[0.0, 0.39215686274509803, 0.0]  IconOffColor=[0.0, 1.0, 0.0]
  Push Button1 : PushButtonBlock  ButtonText=Down  IconOnColor=[0.0, 0.39215686274509803, 0.0]  IconOffColor=[0.0, 1.0, 0.0]
  Push Button2 : PushButtonBlock  ButtonText=Out  IconOnColor=[0.0, 0.39215686274509803, 0.0]  IconOffColor=[0.0, 1.0, 0.0]
  Push Button3 : PushButtonBlock  ButtonText=In  IconOnColor=[0.0, 0.39215686274509803, 0.0]  IconOffColor=[0.0, 1.0, 0.0]
  Push Button4 : PushButtonBlock  ButtonText=L  IconOnColor=[0.0, 0.39215686274509803, 0.0]  IconOffColor=[0.0, 1.0, 0.0]
  Push Button5 : PushButtonBlock  ButtonText=R  IconOnColor=[0.0, 0.39215686274509803, 0.0]  IconOffColor=[0.0, 1.0, 0.0]
  Push Button7 : PushButtonBlock  ButtonText=Down  IconOnColor=[0.0, 0.39215686274509803, 0.0]  IconOffColor=[0.0, 1.0, 0.0]
  Push Button8 : PushButtonBlock  ButtonText=Up  IconOnColor=[0.0, 0.39215686274509803, 0.0]  IconOffColor=[0.0, 1.0, 0.0]
  Subtract BasketR : Sum  Inputs=+-
  Subtract Extend : Sum  Inputs=+-
  Subtract Jib : Sum  Inputs=+-
  Subtract Lift : Sum  Inputs=+-
  Subtract OutAll : Sum  Inputs=+-
  Subtract OutFL : Sum  Inputs=+-
  Subtract OutFR : Sum  Inputs=+-
  Subtract OutRL : Sum  Inputs=+-
  Subtract OutRR : Sum  Inputs=+-
  Subtract Tilt : Sum  Inputs=+-
  Subtract Track : Sum  Inputs=+-
  Subtract Turret : Sum  Inputs=+-
  Sum{1..4} (4 alike) : Sum  Inputs=++|
  Telescope Extend : Constant  Value=0
  Telescope Retract : Constant  Value=0
  Terminator1 : Terminator
  Tilt Down : Constant  Value=0
  Tilt Up : Constant  Value=0
  Track Extend : Constant  Value=0
  Track Retract : Constant  Value=0
  Turret Left : Constant  Value=0
  Turret Right : Constant  Value=0
  Out Bus Element : Outport  PortName=L  Element=Turret
  Out Bus Element1 : Outport  PortName=L  Element=Lift
  Out Bus Element2 : Outport  PortName=L  Element=Tilt
  Out Bus Element3 : Outport  PortName=L  Element=Jib
  Out Bus Element4 : Outport  PortName=L  Element=Extend
  Out Bus Element5 : Outport  PortName=L  Element=BasketR
  Out Bus Element6 : Outport  PortName=L  Element=OutRL
  Out Bus Element7 : Outport  PortName=L  Element=OutFL
  Out Bus Element8 : Outport  PortName=L  Element=TrackL
  Out Bus Element9 : Outport  PortName=L  Element=TrackR
  Out Bus Element10 : Outport  PortName=L  Element=OutRR
  Out Bus Element11 : Outport  PortName=L  Element=OutFR
  L1 : Outport  Port=2
  wires:
  Subtract Track/1 -> Mux/1, Out Bus Element8/1  "TrackL"
  Sum4/1 -> Out Bus Element10/1  "OutRR"
  Sum2/1 -> Out Bus Element11/1  "OutFR"
  Sum3/1 -> Out Bus Element6/1  "OutRL"
  Subtract Jib/1 -> Out Bus Element3/1  "Jib"
  Subtract BasketR/1 -> Out Bus Element5/1  "BasketR"
  Sum1/1 -> Out Bus Element7/1  "OutFL"
  Subtract Tilt/1 -> Out Bus Element2/1  "Tilt"
  Subtract Lift/1 -> Out Bus Element1/1  "Lift"
  Subtract Turret/1 -> Out Bus Element/1  "Turret"
  Subtract Extend/1 -> Out Bus Element4/1  "Extend"
  Lift Up/1 -> Subtract Lift/1  "Up"
  Lift Down/1 -> Subtract Lift/2  "Down"
  S/1 -> Bus Selector/1
  Bus Selector/1 -> L1/1, Terminator1/1  "<Jib Align>"
  Track Retract/1 -> Subtract Track/2  "Retract"
  Track Extend/1 -> Subtract Track/1  "Extend"
  Mux/1 -> Out Bus Element9/1  "TrackR"
  Turret Right/1 -> Subtract Turret/2  "Right"
  Turret Left/1 -> Subtract Turret/1  "Left"
  Tilt Up/1 -> Subtract Tilt/1  "Up"
  Tilt Down/1 -> Subtract Tilt/2  "Down"
  Telescope Retract/1 -> Subtract Extend/2  "Retract"
  Telescope Extend/1 -> Subtract Extend/1  "Extend"
  Basket Left/1 -> Subtract BasketR/1  "Left"
  Basket Right/1 -> Subtract BasketR/2  "Right"
  Jib Retract/1 -> Subtract Jib/2  "Retract"
  Jib Extend/1 -> Subtract Jib/1  "Extend"
  OutFL Extend/1 -> Subtract OutFL/1  "Extend"
  OutFL Retract1/1 -> Subtract OutFL/2  "Retract"
  OutFR Retract/1 -> Subtract OutFR/2  "Retract"
  OutFR Extend/1 -> Subtract OutFR/1  "Extend"
  Subtract OutFR/1 -> Sum2/2
  Subtract OutFL/1 -> Sum1/2
  OutRL Extend/1 -> Subtract OutRL/1  "Extend"
  OutRL Retract1/1 -> Subtract OutRL/2  "Retract"
  Subtract OutRL/1 -> Sum3/2
  OutRR Retract/1 -> Subtract OutRR/2  "Retract"
  OutRR Extend/1 -> Subtract OutRR/1  "Extend"
  Subtract OutRR/1 -> Sum4/2
  OutAll Retract/1 -> Subtract OutAll/2  "Retract"
  OutAll Extend/1 -> Subtract OutAll/1  "Extend"
  Subtract OutAll/1 -> Sum4/1, Sum3/1, Sum2/1, Sum1/1
